simulink model "FinalProject_Transmitter"  (R2023b)
settings: Solver=FixedStepAuto  StartTime=0.0  StopTime=inf  FixedStep=0.01  RelTol=1e-3  EnableMultiTasking=on
libraries: arduinolib x7, slpidlib x1, arduinosensorlib x1
settings Model: ExtModeTrigDuration=2  Creator=20210798  LastModifiedBy=20210798
settings OptimizationCC: EnhancedBackFolding=on  PassReuseOutputArgsAs=Individual arguments  ZeroExternalMemoryAtStartup=off  ZeroInternalMemoryAtStartup=off  MaxStackSize=64  OptimizeBlockOrder=speed  DifferentSizesBufferReuse=on  OptimizationCustomize=off  EfficientTunableParamExpr=on
settings DebuggingCC: ParameterTunabilityLossMsg=error
settings HardwareCC: ProdBitPerInt=16  ProdBitPerPointer=16  ProdBitPerSizeT=16  ProdBitPerPtrDiffT=16  ProdLargestAtomicFloat=None  ProdWordSize=8  ProdHWDeviceType=Atmel->AVR  UseEmbeddedCoderFeatures=off  UseSimulinkCoderFeatures=off
settings SFSimCC: MATLABDynamicMemAlloc=off
settings RTWCC: Description=Embedded Coder  SystemTargetFile=ert.tlc  HardwareBoard=Arduino Uno  TemplateMakefile=ert_default_tmf  Toolchain=Arduino AVR  BuildConfiguration=Faster Runs
settings CodeAppCC: ForceParamTrailComments=on  IgnoreCustomStorageClasses=off  OperatorAnnotations=on  SimulinkDataObjDesc=on  SFDataObjDesc=on  MangleLength=10  InsertBlockDesc=on
settings ERTTargetCC: SupportContinuousTime=on  SupportNonInlinedSFcns=on  SupportVariableSizeSignals=on  ExtModeTransport=3  ExtModeStaticAlloc=on  ExtModeAutomaticAllocSize=off  ExtModeStaticAllocSize=250  ExtModeMexFile=ext_xcp  ExtModeIntrfLevel=Level2 - Open

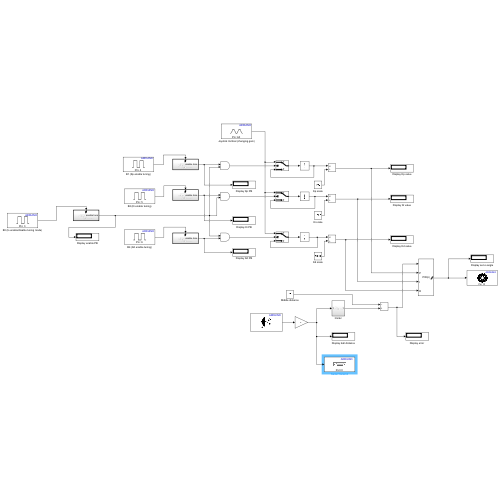
[thumbnail: Simulink's stored preview of the top-level diagram]
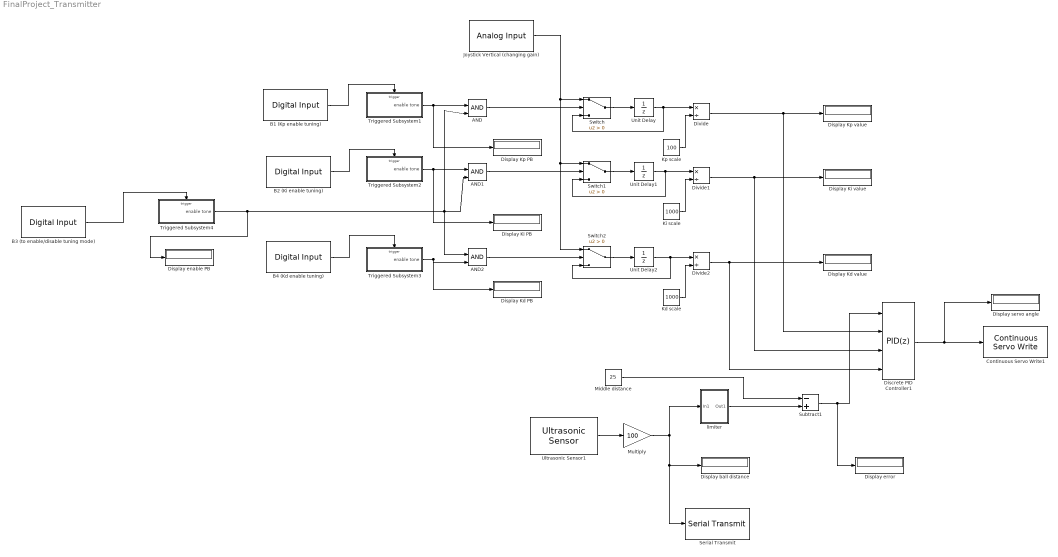
== system FinalProject_Transmitter ==
  AND : Logic  IconShape=distinctive  AllPortsSameDT=off  OutDataTypeStr=boolean
  AND1 : Logic  IconShape=distinctive  AllPortsSameDT=off  OutDataTypeStr=boolean
  AND2 : Logic  IconShape=distinctive  AllPortsSameDT=off  OutDataTypeStr=boolean
  B1 (Kp enable tuning) : arduinolib/Digital Input  pinNumber=4  mode=Default  Direction=input  SampleTime=0.1  blockPlatform=arduino
  B2 (Ki enable tuning) : arduinolib/Digital Input  pinNumber=5  mode=Default  Direction=input  SampleTime=0.1  blockPlatform=arduino
  B3 (to enable/disable tuning mode) : arduinolib/Digital Input  pinNumber=3  mode=Default  Direction=input  SampleTime=0.1  blockPlatform=arduino
  B4 (Kd enable tuning) : arduinolib/Digital Input  pinNumber=6  mode=Default  Direction=input  SampleTime=0.1  blockPlatform=arduino
  Continuous Servo Write1 : arduinolib/Continuous Servo Write  pinNumber=10  ServoIndex=0  blockPlatform=ARDUINO
  Discrete PID Controller1 : slpidlib/PID Controller  Controller=PID  Form=Parallel  TimeDomain=Discrete-time  UseExternalTs=off  SampleTime=-1  IntegratorMethod=Forward Euler  FilterMethod=Forward Euler  ControllerParametersSource=external  P=2  I=0.17  UseKiTs=off  D=0.023  N=50  UseFilter=off  TunerSelectOption=Transfer Function Based (PID Tuner App)  InitialConditionSource=internal  InitialConditionForIntegrator=0  InitialConditionForFilter=0  DifferentiatorICPrevScaledInput=0  ExternalReset=none  TrackingMode=off  Kt=1  LimitOutput=on  SatLimitsSource=internal  UpperSaturationLimit=75  LowerSaturationLimit=-90  LinearizeAsGain=off  AntiWindupMode=none  Kb=1  LimitIntegrator=off  UpperIntegratorSaturationLimit=inf  LowerIntegratorSaturationLimit=-inf  RndMeth=Round  POutMin=[]  POutMax=[]  IOutMin=[]  IOutMax=[]  DOutMin=[]  DOutMax=[]  NOutMin=[]  NOutMax=[]  SumOutMin=[]  SumOutMax=[]  SaturationOutMin=[]  SaturationOutMax=[]  PParamMin=[]  PParamMax=[]  IParamMin=[]  IParamMax=[]  DParamMin=[]  DParamMax=[]  NParamMin=[]  NParamMax=[]  KbParamMin=[]  KbParamMax=[]  KtParamMin=[]  KtParamMax=[]  KbOutMin=[]  KbOutMax=[]  KtOutMin=[]  KtOutMax=[]  IntegratorOutMin=[]  IntegratorOutMax=[]  FilterOutMin=[]  FilterOutMax=[]  SumI1OutMin=[]  SumI1OutMax=[]  SumI2OutMin=[]  SumI2OutMax=[]  SumI3OutMin=[]  SumI3OutMax=[]  SumI4OutMin=[]  SumI4OutMax=[]  SumDOutMin=[]  SumDOutMax=[]  DifferentiatorOutMin=[]  DifferentiatorOutMax=[]  FilterDiffOutCoefMin=[]  FilterDiffOutCoefMax=[]  ReciprocalOutMin=[]  ReciprocalOutMax=[]  SumDenOutMin=[]  SumDenOutMax=[]  SumNumOutMin=[]  SumNumOutMax=[]  DivideOutMin=[]  DivideOutMax=[]  UdiffTsProdOutMin=[]  UdiffTsProdOutMax=[]  NTsProdOutMin=[]  NTsProdOutMax=[]  UintegralTsProdOutMin=[]  UintegralTsProdOutMax=[]  UngainTsProdOutMin=[]  UngainTsProdOutMax=[]  ClampingZeroOutDataTypeStr=Inherit: Inherit via back propagation  ClampingZeroOutMin=[]  ClampingZeroOutMax=[]  FilterDenConstantOutDataTypeStr=Inherit: Inherit via back propagation  FilterDenConstantOutMin=[]  FilterDenConstantOutMax=[]  PCopyOutDataTypeStr=Inherit: Inherit via back propagation  PCopyOutMin=[]  PCopyOutMax=[]  NCopyOutDataTypeStr=Inherit: Inherit via back propagation  NCopyOutMin=[]  NCopyOutMax=[]  IntegratorContinuousStateAttributes=''  IntegratorStateMustResolveToSignalObject=off  IntegratorRTWStateStorageClass=Auto  FilterContinuousStateAttributes=''  FilterStateMustResolveToSignalObject=off  FilterRTWStateStorageClass=Auto  ParallelPVariant=ExternalParameters  IdealPVariant=Disabled  IVariant=ExternalParameters  DVariant=ExternalParameters  IntegratorVariant=Discrete  SatVariant=Enabled  AWVariant=Passthrough  PCopyVariant=Disabled  TRVariant=Disabled  FdbkBlocksVariant=Forward  IdealPFdbkVariant=Disabled  SatFdbkVariant=Disabled  DerivativeFilterVariant=Differentiator  NVariant=Passthrough  NCopyVariant=Disabled_SignalSpec  FilterICVariant=InternalICsDifferentiator  IntegratorICVariant=InternalICs  ExternalResetVariant=Disabled  TRSumVariant=Passthrough  SumFdbkVariant=Disabled  SumVariant=Sum_PID  TsampFilterVariant=InternalTs  TsampNgainVariant=Passthrough  TsampIntegralVariant=Disabled_SignalSpec  ExternalSaturationOutDataTypeStr=Inherit: Same as second input
  Display Kd PB : Display
  Display Kd value : Display
  Display Ki PB : Display
  Display Ki value : Display
  Display Kp PB : Display
  Display Kp value : Display
  Display ball distance : Display
  Display enable PB : Display
  "Display error " : Display
  Display servo angle : Display
  Divide : Product  Inputs=*/
  Divide1 : Product  Inputs=*/
  Divide2 : Product  Inputs=*/
  Joystick Vertical (changing gain) : arduinolib/Analog Input  pinNumber=0  ReadResultsOnly=off  ConversionTriggerSource=Software  ExternalTriggerType=uint32( 0 )  OutputDataType=uint16  EnableConversionCompleteNotify=off  EnableOuputStatus=off  SampleTime=-1  blockPlatform=arduino
  Kd scale : Constant  Value=1000
  Ki scale : Constant  Value=1000
  Kp scale : Constant  Value=100
  Middle distance : Constant  Value=25
  Multiply : Gain  Gain=100
  Serial Transmit : arduinolib/Serial Transmit  portNumber=0  sendmode=write  sendformat=Decimal  floatprecision=2  blockPlatform=arduino
  Subtract1 : Sum  Inputs=-+
  Switch : Switch  Criteria=u2 > Threshold  SaturateOnIntegerOverflow=off  InputSameDT=off
  Switch1 : Switch  Criteria=u2 > Threshold  SaturateOnIntegerOverflow=off  InputSameDT=off
  Switch2 : Switch  Criteria=u2 > Threshold  SaturateOnIntegerOverflow=off  InputSameDT=off
  Triggered Subsystem1 : Subsystem  TreatAsAtomicUnit=on
  Triggered Subsystem2 : Subsystem  TreatAsAtomicUnit=on
  Triggered Subsystem3 : Subsystem  TreatAsAtomicUnit=on
  Triggered Subsystem4 : Subsystem  TreatAsAtomicUnit=on
  Ultrasonic Sensor1 : arduinosensorlib/Ultrasonic Sensor  NumSignalPins=2  TrigPin=8  EchoPin=9  SignalPin=3  SampleTime_=0.1  blockPlatform=ARDUINO
  Unit Delay : UnitDelay  SampleTime=-1  HasFrameUpgradeWarning=on
  Unit Delay1 : UnitDelay  SampleTime=-1  HasFrameUpgradeWarning=on
  Unit Delay2 : UnitDelay  SampleTime=-1  HasFrameUpgradeWarning=on
  limiter : Subsystem
  wires:
  Middle distance/1 -> Subtract1/1
  Ki scale/1 -> Divide1/2
  Divide/1 -> Display Kp value/1, Discrete PID Controller1/2
  Divide1/1 -> Discrete PID Controller1/3, Display Ki value/1
  Kp scale/1 -> Divide/2
  Ultrasonic Sensor1/1 -> Multiply/1
  Kd scale/1 -> Divide2/2
  Divide2/1 -> Discrete PID Controller1/4, Display Kd value/1
  limiter/1(Out1) -> Subtract1/2
  Subtract1/1 -> "Display error "/1, Discrete PID Controller1/1
  Discrete PID Controller1/1 -> Display servo angle/1, Continuous Servo Write1/1
  Multiply/1 -> Serial Transmit/1, Display ball distance/1, limiter/1(In1)
  B3 (to enable/disable tuning mode)/1 -> Triggered Subsystem4/Trigger
  B4 (Kd enable tuning)/1 -> Triggered Subsystem3/Trigger
  B2 (Ki enable tuning)/1 -> Triggered Subsystem2/Trigger
  B1 (Kp enable tuning)/1 -> Triggered Subsystem1/Trigger
  Triggered Subsystem1/1(enable tone) -> Display Kp PB/1, AND/1
  Triggered Subsystem3/1(enable tone) -> Display Kd PB/1, AND2/2
  Triggered Subsystem2/1(enable tone) -> Display Ki PB/1, AND1/1
  Triggered Subsystem4/1(enable tone) -> Display enable PB/1, AND2/1, AND1/2, AND/2
  AND/1 -> Switch/2
  AND2/1 -> Switch2/2
  AND1/1 -> Switch1/2
  Joystick Vertical (changing gain)/1 -> Switch2/1, Switch1/1, Switch/1
  Unit Delay/1 -> Switch/3, Divide/1
  Switch/1 -> Unit Delay/1
  Unit Delay1/1 -> Switch1/3, Divide1/1
  Switch1/1 -> Unit Delay1/1
  Unit Delay2/1 -> Switch2/3, Divide2/1
  Switch2/1 -> Unit Delay2/1

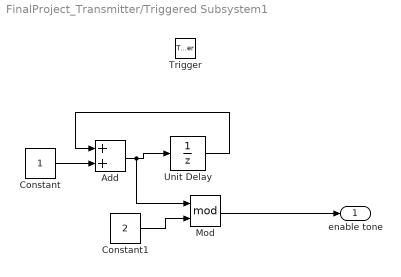
== system FinalProject_Transmitter/Triggered Subsystem1 ==
  Trigger : TriggerPort  VariantControl=(inherit)
  Add : Sum
  Constant : Constant
  Constant1 : Constant  Value=2
  Mod : Math  Operator=mod
  Unit Delay : UnitDelay  SampleTime=-1  HasFrameUpgradeWarning=on
  enable tone : Outport
  wires:
  Mod/1 -> enable tone/1
  Constant/1 -> Add/2
  Constant1/1 -> Mod/2
  Add/1 -> Mod/1, Unit Delay/1
  Unit Delay/1 -> Add/1

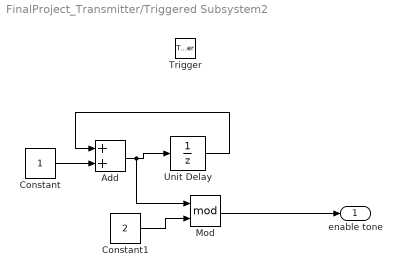
== system FinalProject_Transmitter/Triggered Subsystem2 ==
  Trigger : TriggerPort  VariantControl=(inherit)
  Add : Sum
  Constant : Constant
  Constant1 : Constant  Value=2
  Mod : Math  Operator=mod
  Unit Delay : UnitDelay  SampleTime=-1  HasFrameUpgradeWarning=on
  enable tone : Outport
  wires:
  Mod/1 -> enable tone/1
  Constant/1 -> Add/2
  Constant1/1 -> Mod/2
  Add/1 -> Mod/1, Unit Delay/1
  Unit Delay/1 -> Add/1

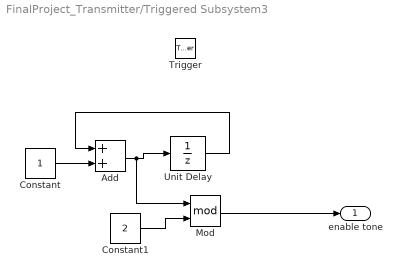
== system FinalProject_Transmitter/Triggered Subsystem3 ==
  Trigger : TriggerPort  VariantControl=(inherit)
  Add : Sum
  Constant : Constant
  Constant1 : Constant  Value=2
  Mod : Math  Operator=mod
  Unit Delay : UnitDelay  SampleTime=-1  HasFrameUpgradeWarning=on
  enable tone : Outport
  wires:
  Mod/1 -> enable tone/1
  Constant/1 -> Add/2
  Constant1/1 -> Mod/2
  Add/1 -> Mod/1, Unit Delay/1
  Unit Delay/1 -> Add/1

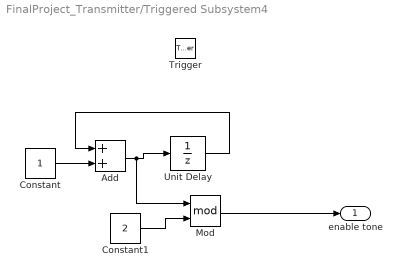
== system FinalProject_Transmitter/Triggered Subsystem4 ==
  Trigger : TriggerPort  VariantControl=(inherit)
  Add : Sum
  Constant : Constant
  Constant1 : Constant  Value=2
  Mod : Math  Operator=mod
  Unit Delay : UnitDelay  SampleTime=-1  HasFrameUpgradeWarning=on
  enable tone : Outport
  wires:
  Mod/1 -> enable tone/1
  Constant/1 -> Add/2
  Constant1/1 -> Mod/2
  Add/1 -> Mod/1, Unit Delay/1
  Unit Delay/1 -> Add/1

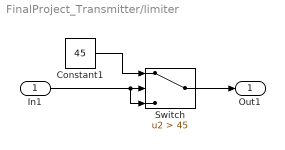
== system FinalProject_Transmitter/limiter ==
  In1 : Inport
  Constant1 : Constant  Value=45
  Switch : Switch  Criteria=u2 > Threshold  Threshold=45  SaturateOnIntegerOverflow=off  InputSameDT=off
  Out1 : Outport
  wires:
  Switch/1 -> Out1/1
  In1/1 -> Switch/3, Switch/2
  Constant1/1 -> Switch/1
